simulink model "LCK"  (R2020b)
settings: Solver=FixedStepAuto  StartTime=0.0  StopTime=Inf  RelTol=1e-3
PostLoadFcn:
  | if any(exist('dsrtsu_mdlpostloadfcn', 'file') ~= 0), dsrtsu_mdlpostloadfcn('Execute', bdroot); end
InitFcn:
  | , if any(exist('dsmpb_private', 'file') ~= 0), dsmpb_private('dsmpb_mdlclblib', 'Init', bdroot); end,
PreSaveFcn:
  | , if any(exist('dsmpb_private', 'file') ~= 0), dsmpb_private('dsmpb_mdlclblib', 'PreSave', bdroot); end,
CloseFcn:
  | , if any(exist('dsmpb_private', 'file') ~= 0), dsmpb_private('dsmpb_mdlclblib', 'Close', bdroot); end,
settings Model: DataDictionary=HWA_DDs.sldd  RTICANMMDATA=struct('GeneralSetupData',struct('modelroot','F:\ADAS_Store\ADAS_Store\Adas\VSM\LSSState\LCK','generalsettings',struct('filesettings',struct('destfolder',struct('Name','RTICANMM_FILES','Check',1),'buildfolder',struct('Name','.','Check',1),'AbsDestfolder',struct('Name','F:\ADAS_Store\ADAS_Store\Adas\VSM\LSSState\LCK\RTICANMM_FILES'),'AbsBuildfolder',struct('Name','F:\ADAS_Store\ADAS_Store\Adas\VSM\LSSState\LCK'))),'options',struct('addpaths',1,'rmpaths',1,'addtrcexclusion',false,'cannavigator',struct('checkmonitoring',0),'show_usrtrc',0,'use_usrtrc',0),'advanced',struct('options',ones(1,100)),'MPSetup',{{}},'RTI',struct('Type','DSRT','Ver','4.2','Date','02-Nov-2019'),'modelname','LCK','block','LCK'))  DSRTSU_INTERNAL_RTIFPGA=150  Creator=GW00199575  LastModifiedBy=GW00199575
settings OptimizationCC: BlockReduction=off  ConditionallyExecuteInputs=off  OptimizeBlockIOStorage=off  BufferReuse=off
settings DebuggingCC: TasksWithSamePriorityMsg=none
settings HardwareCC: ProdBitPerPointer=32  ProdBitPerSizeT=32  ProdBitPerPtrDiffT=32  ProdLargestAtomicInteger=Integer  ProdWordSize=32  ProdHWDeviceType=Custom Processor->Custom
settings ModelReferenceCC: EnableParallelModelReferenceBuilds=on  ModelReferenceNumInstancesAllowed=Single
settings SFSimCC: MATLABDynamicMemAlloc=off
settings RTWCC: Description=dSPACE Run-Time Target (for VEOS on Windows and ConfigurationDesk)  SystemTargetFile=dsrt.tlc  GenCodeOnly=on  MakeCommand=make_dsrt  TemplateMakefile=dsrt_default_tmf  RTWVerbose=off
settings CodeAppCC: MaxIdLength=128
settings STFCustomTargetCC: TargetLangStandard=C99 (ISO)  ParMdlRefBuildCompliant=on  ConcurrentExecutionCompliant=off  CPPClassGenCompliant=off  GRTInterface=off  SystemTargetFile=dsrt.tlc
settings GRTTargetCC: CompOptLevelCompliant=off  ConcurrentExecutionCompliant=off  CombineOutputUpdateFcns=off  MatFileLogging=off  CPPClassGenCompliant=off  UseToolchainInfoCompliant=off

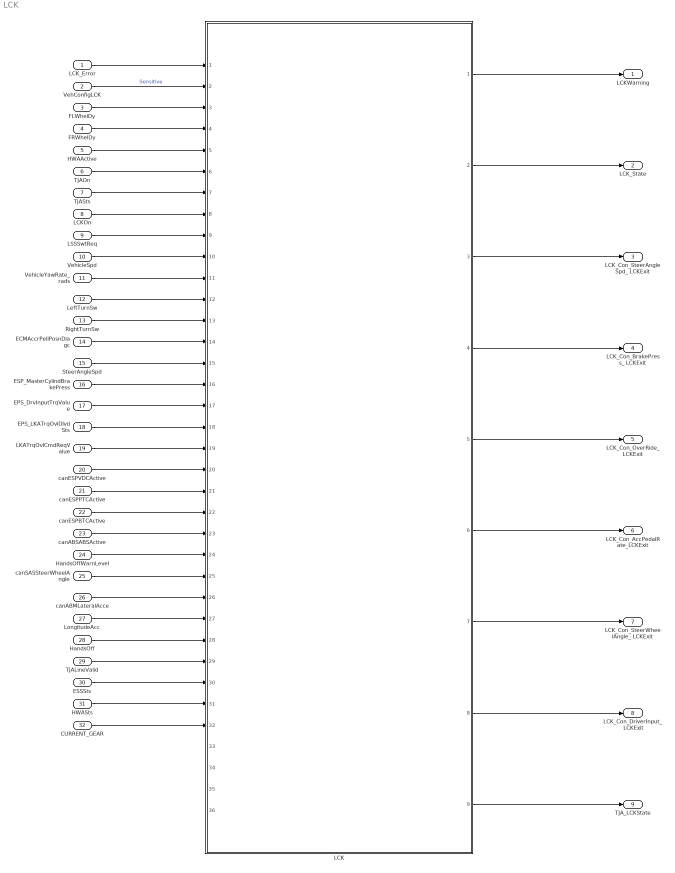
== system LCK ==
  LCK_Error : Inport  OutDataTypeStr=boolean
  VehConfigLCK : Inport  Port=2  OutDataTypeStr=uint8
  FLWhelDy : Inport  Port=3  OutDataTypeStr=single
  FRWhelDy : Inport  Port=4  OutDataTypeStr=single
  HWAActive : Inport  Port=5  OutDataTypeStr=boolean
  TJAOn : Inport  Port=6  OutDataTypeStr=boolean
  TJASts : Inport  Port=7  OutDataTypeStr=uint8
  LCKOn : Inport  Port=8
  LSSSwtReq : Inport  Port=9
  VehicleSpd : Inport  Port=10  OutDataTypeStr=single
  VehicleYawRate_rads : Inport  Port=11  OutDataTypeStr=single
  LeftTurnSw : Inport  Port=12  OutDataTypeStr=boolean
  RightTurnSw : Inport  Port=13  OutDataTypeStr=boolean
  ECMAccrPellPosnDiagc : Inport  Port=14  OutDataTypeStr=single
  SteerAngleSpd : Inport  Port=15  OutDataTypeStr=single
  ESP_MasterCylindBrakePress : Inport  Port=16  OutDataTypeStr=single
  EPS_DrvInputTrqValue : Inport  Port=17  OutDataTypeStr=single
  EPS_LKATrqOvlDlvdSts : Inport  Port=18  OutDataTypeStr=uint8
  LKATrqOvlCmdReqValue : Inport  Port=19  OutDataTypeStr=single
  canESPVDCActive : Inport  Port=20  OutDataTypeStr=boolean
  canESPPTCActive : Inport  Port=21  OutDataTypeStr=boolean
  canESPBTCActive : Inport  Port=22  OutDataTypeStr=boolean
  canABSABSActive : Inport  Port=23  OutDataTypeStr=boolean
  HandsOffWarnLevel : Inport  Port=24  OutDataTypeStr=uint8
  canSASSteerWheelAngle : Inport  Port=25  OutDataTypeStr=single
  canABMLateralAcce : Inport  Port=26  OutDataTypeStr=single
  LongitudeAcc : Inport  Port=27  OutDataTypeStr=single
  HandsOff : Inport  Port=28  OutDataTypeStr=boolean
  TJALineValid : Inport  Port=29  OutDataTypeStr=boolean
  ESSSts : Inport  Port=30  OutDataTypeStr=uint8
  HWASts : Inport  Port=31  OutDataTypeStr=uint8
  CURRENT_GEAR : Inport  Port=32  OutDataTypeStr=uint8
  LCK : Subsystem  ReferencedSubsystem=PvtSubSys_VSM_LCK
  LCKWarning : Outport
  LCK_State : Outport  Port=2
  LCK_Con_SteerAngleSpd_ LCKExit : Outport  Port=3
  LCK_Con_BrakePress_ LCKExit : Outport  Port=4
  LCK_Con_OverRide_ LCKExit : Outport  Port=5
  LCK_Con_AccPedalRate_LCKExit : Outport  Port=6
  LCK_Con_SteerWheelAngle_ LCKExit : Outport  Port=7
  LCK_Con_DriverInput_ LCKExit : Outport  Port=8
  TJA_LCKState : Outport  Port=9
  wires:
  LCK_Error/1 -> LCK/1
  VehConfigLCK/1 -> LCK/2  "Sensitive"
  FLWhelDy/1 -> LCK/3
  FRWhelDy/1 -> LCK/4
  HWAActive/1 -> LCK/5
  LCK/1 -> LCKWarning/1
  LCK/2 -> LCK_State/1
  LCK/9 -> TJA_LCKState/1
  LCK/3 -> LCK_Con_SteerAngleSpd_ LCKExit/1
  LCK/4 -> LCK_Con_BrakePress_ LCKExit/1
  LCK/5 -> LCK_Con_OverRide_ LCKExit/1
  LCK/6 -> LCK_Con_AccPedalRate_LCKExit/1
  LCK/7 -> LCK_Con_SteerWheelAngle_ LCKExit/1
  LCK/8 -> LCK_Con_DriverInput_ LCKExit/1
  TJAOn/1 -> LCK/6
  TJASts/1 -> LCK/7
  LCKOn/1 -> LCK/8
  LSSSwtReq/1 -> LCK/9
  VehicleSpd/1 -> LCK/10
  VehicleYawRate_rads/1 -> LCK/11
  LeftTurnSw/1 -> LCK/12
  RightTurnSw/1 -> LCK/13
  ECMAccrPellPosnDiagc/1 -> LCK/14
  SteerAngleSpd/1 -> LCK/15
  ESP_MasterCylindBrakePress/1 -> LCK/16
  EPS_DrvInputTrqValue/1 -> LCK/17
  EPS_LKATrqOvlDlvdSts/1 -> LCK/18
  LKATrqOvlCmdReqValue/1 -> LCK/19
  canESPVDCActive/1 -> LCK/20
  canESPPTCActive/1 -> LCK/21
  canESPBTCActive/1 -> LCK/22
  canABSABSActive/1 -> LCK/23
  HandsOffWarnLevel/1 -> LCK/24
  canSASSteerWheelAngle/1 -> LCK/25
  canABMLateralAcce/1 -> LCK/26
  LongitudeAcc/1 -> LCK/27
  HandsOff/1 -> LCK/28
  TJALineValid/1 -> LCK/29
  ESSSts/1 -> LCK/30
  HWASts/1 -> LCK/31
  CURRENT_GEAR/1 -> LCK/32
